simulink model "PenduloSK"  (R2024a)
settings: Solver=ode4  StartTime=0.0  StopTime=Tsim  FixedStep=Ts  RelTol=1e-3
values from neighbouring files (symbols this model uses):
  DeltaTd = 0.25    [PeduloInvertido.m]
  Fd = 0.1    [PeduloInvertido.m]
  g = 9.81    [PeduloInvertido.m]
  k = 0.15    [PeduloInvertido.m]
  l = 0.2    [PeduloInvertido.m]
  m1 = 0.2    [PeduloInvertido.m]
  m2 = 0.1    [PeduloInvertido.m]
  Td = 2    [PeduloInvertido.m]
  x0 = [0;pi;0;0]    [PeduloInvertido.m]
libraries: vrlib x3
settings Model: Creator=andre  LastModifiedBy=andre

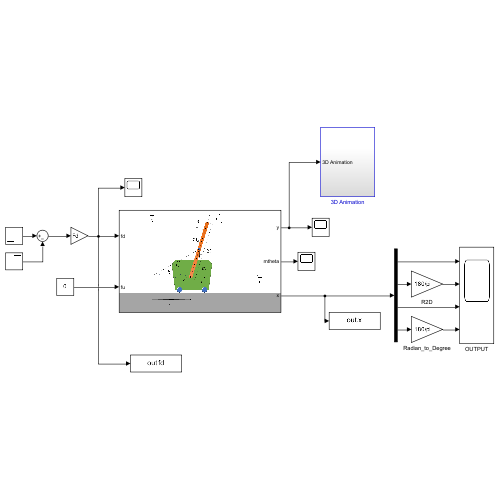
[thumbnail: Simulink's stored preview of the top-level diagram]
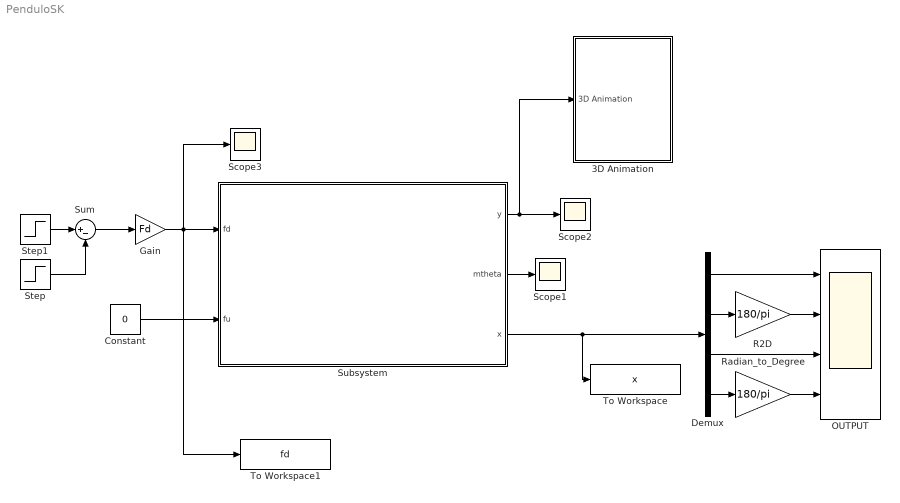
== system PenduloSK ==
  3D Animation : Subsystem
  Constant : Constant  Value=0
  Demux : Demux
  Gain : Gain  Gain=Fd
  OUTPUT : Scope  NumInputPorts=4
  R2D : Gain  Gain=180/pi
  Radian_to_Degree : Gain  Gain=180/pi
  Scope1 : Scope
  Scope2 : Scope
  Scope3 : Scope
  Step : Step  Time=Td+DeltaTd  SampleTime=0
  Step1 : Step  Time=Td  SampleTime=0
  Subsystem : Subsystem
      mask Display: image('PenduloInvertido.png');
  Sum : Sum  Inputs=|+-
  To Workspace : ToWorkspace  VariableName=x  SampleTime=-1
  To Workspace1 : ToWorkspace  VariableName=fd  SampleTime=-1
  wires:
  Constant/1 -> Subsystem/2(fu)
  Subsystem/2(mtheta) -> Scope1/1
  Subsystem/1(y) -> 3D Animation/1(3D Animation), Scope2/1
  Step/1 -> Sum/2
  Step1/1 -> Sum/1
  Sum/1 -> Gain/1
  Gain/1 -> To Workspace1/1, Scope3/1, Subsystem/1(fd)
  Radian_to_Degree/1 -> OUTPUT/4
  Demux/1 -> OUTPUT/1
  R2D/1 -> OUTPUT/2
  Demux/3 -> OUTPUT/3
  Demux/4 -> Radian_to_Degree/1
  Demux/2 -> R2D/1
  Subsystem/3(x) -> To Workspace/1, Demux/1

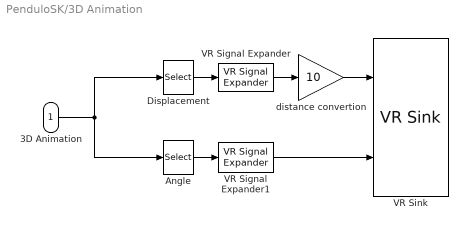
== system PenduloSK/3D Animation ==
  3D Animation : Inport
  Angle : Selector  InputPortWidth=2  IndexOptions=Index vector (dialog)  Indices=[2]  OutputSizes=1
  Displacement : Selector  InputPortWidth=2  IndexOptions=Index vector (dialog)  Indices=[1]  OutputSizes=1
  VR Signal Expander : vrlib/VR Signal Expander  outwidth=3  outidx=[1]
  VR Signal Expander1 : vrlib/VR Signal Expander  outwidth=4  outidx=[4]
  VR Sink : vrlib/VR Sink  InstantiateOnLoad=on  SampleTime=0.02  ViewEnable=on  RemoteChange=off  RemoteView=off  FieldsWritten=cart.translation.3.1.1.double#joint.rotation.4.1.1.double  WorldFileName=Inverted_pendulum12.wrl  AutoView=off  VideoDimensions=[]  AllowVariableSize=off
  distance convertion : Gain  Gain=10
  wires:
  VR Signal Expander/1 -> distance convertion/1
  3D Animation/1 -> Angle/1, Displacement/1
  Displacement/1 -> VR Signal Expander/1
  Angle/1 -> VR Signal Expander1/1
  VR Signal Expander1/1 -> VR Sink/2
  distance convertion/1 -> VR Sink/1

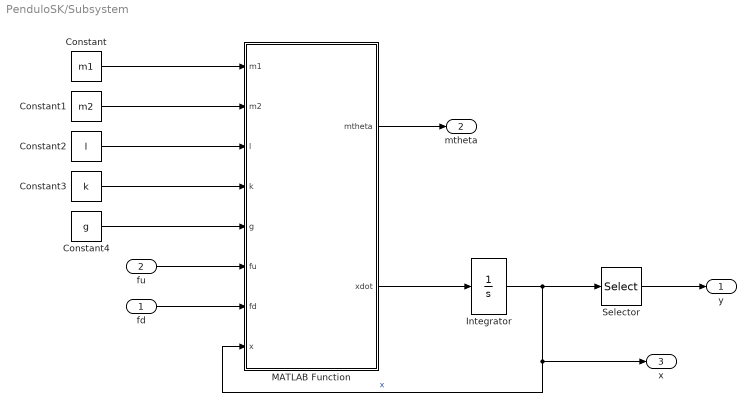
== system PenduloSK/Subsystem ==
  fd : Inport
  fu : Inport  Port=2
  Constant : Constant  Value=m1
  Constant1 : Constant  Value=m2
  Constant2 : Constant  Value=l
  Constant3 : Constant  Value=k
  Constant4 : Constant  Value=g
  Integrator : Integrator  InitialCondition=x0
  MATLAB Function : MATLAB Function  TreatAsAtomicUnit=on
  Selector : Selector  InputPortWidth=4  IndexOptions=Index vector (dialog)  Indices=[1 2]  OutputSizes=1
  y : Outport
  mtheta : Outport  Port=2
  x : Outport  Port=3
  wires:
  Selector/1 -> y/1
  Integrator/1 -> Selector/1, x/1, MATLAB Function/8(x)  "x"
  Constant4/1 -> MATLAB Function/5(g)
  fu/1 -> MATLAB Function/6(fu)
  fd/1 -> MATLAB Function/7(fd)
  Constant/1 -> MATLAB Function/1(m1)
  Constant1/1 -> MATLAB Function/2(m2)
  Constant3/1 -> MATLAB Function/4(k)
  MATLAB Function/2(xdot) -> Integrator/1
  Constant2/1 -> MATLAB Function/3(l)
  MATLAB Function/1(mtheta) -> mtheta/1

== matlab function PenduloSK/Subsystem/MATLAB Function ==
  data: mtheta output; m1 input; xdot output; m2 input; l input; k input; g input; fu input; fd input; x input
function [mtheta,xdot] = fcn(m1,m2,l,k,g,fu,fd,x)
    %% Se desempaquetan las variables de estado
    y=x(1);
    theta=x(2);
    vy=x(3);
    omega=x(4);
    %% Se crean los Parametros Intermendios del Modelo
    Jb=(4/3)*m2*l^2;
    mtheta=m1+m2*(1-(3/4)*cos(theta)^2);
    %% Se calculan las Derivadas mediante f(x,u)
    xdot=zeros(4,1);
    xdot(1) = vy ; %% Se calcula la derivada de y 
    xdot(2) = omega; %% Se calcula la derivada de theta
    xdot(3) = (fu+fd-k*y+sin(theta)*l*m2*omega^2)/mtheta-(g*((m2)^2)*(l^2)*sin(theta)*cos(theta)+2*fd*m2*(l^2)*cos(theta)^2)/(Jb*mtheta); %% se calcula la derivada de vy
    xdot(4) = ((m1+m2)/(Jb*mtheta))*(2*fd*l*cos(theta)+g*m2*l*sin(theta))-((m2*l*cos(theta))/(Jb*mtheta))*(m2*l*sin(theta)*omega^2 +fd+fu-k*y); %% se calcula la derivada de omega
end
